simulink model "ROSCO"  (R2023a)
settings: Solver=ode4  StartTime=0.0  StopTime=TMax  FixedStep=simu.dt  RelTol=1e-3  EnableMultiTasking=on
undefined symbols (not defined in the file): A_total, Azimuth_list, B_total, Bd_total, C_total, D_total, Dd_total, DiscIntNeverNeededParam, F, n_FixFrameInputs, n_FixFrameOutputs, n_FixFrameStates2, n_RotTripletInputs, n_RotTripletOutputs, n_RotTripletStates2, new_seq_inp, new_seq_out, new_seq_states, OutList, Parameter, R, rpm2radps, simu, strmatch, uop_total, windspeed_list, wop_total, xop_total, yop_List_total
libraries: simulink x10
(part 1 of 5)
settings Model: Creator=nabbas  LastModifiedBy=16708
settings SolverCC: AlgebraicLoopSolver=TrustRegion
settings DataIOCC: SaveTime=off  ReturnWorkspaceOutputs=off  SignalLoggingName=sigsOut
settings DebuggingCC: UnconnectedInputMsg=warning  UnconnectedOutputMsg=warning  UnconnectedLineMsg=warning  ArithmeticOperatorsInVariantConditions=warning
settings ModelReferenceCC: EnableRefExpFcnMdlSchedulingChecks=on
settings SFSimCC: SimUseLocalCustomCode=off  CustomCodeUndefinedFunction=UseInterfaceOnly
settings RTWCC: RTWUseLocalCustomCode=off
settings CodeAppCC: StateflowObjectComments=on

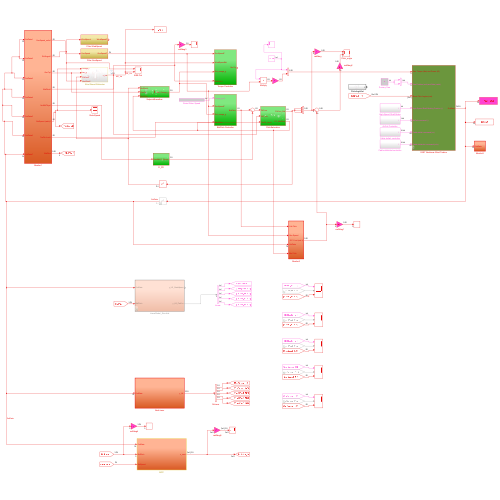
[thumbnail: Simulink's stored preview of the top-level diagram]
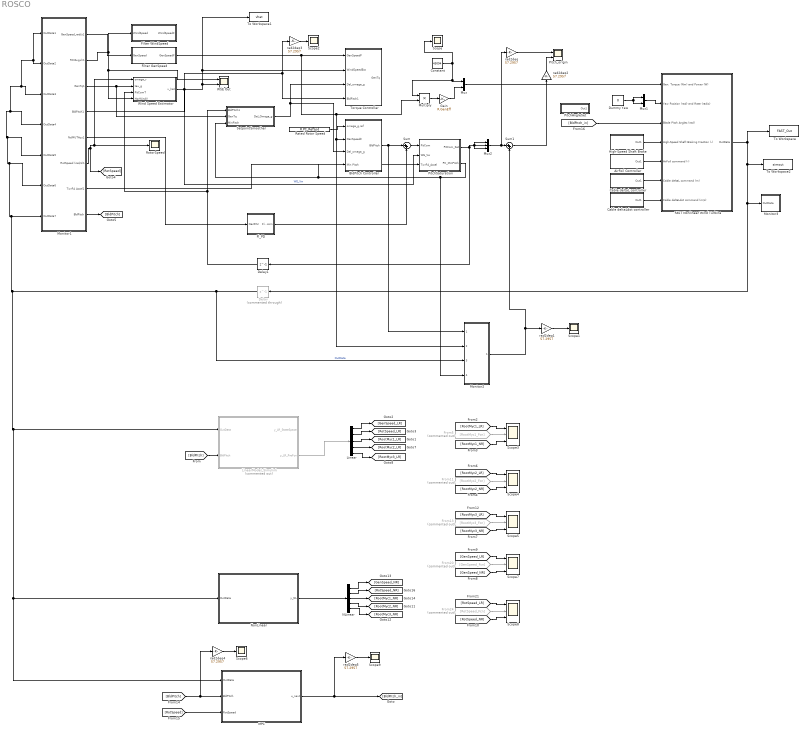
== system ROSCO ==
  AirFoil Controller : Subsystem
  BldPitch Controller : Subsystem
  Cable deltaL controller : Subsystem
  Cable deltaLdot controller : Subsystem
  Constant : Constant  Value=43094
  Delay : Delay  Commented=through  DelayLength=1
  Delay1 : Delay  DelayLength=1
  Dummy Yaw : Constant  Value=0
  FAST Nonlinear Wind Turbine : Subsystem  mask(FAST Nonlinear Wind Turbine){}
      mask help: This block contains the FAST S-Function.
      mask init:
      | clear FAST_SFunc
  Filter GenSpeed : Subsystem
  Filter WindSpeed : Subsystem
  Fl_PD : Subsystem
  From11 : From  Commented=on  GotoTag=RootMyc2_Fcn
  From13 : From  Commented=on  GotoTag=RootMyc3_Fcn
  From20 : From  Commented=on  GotoTag=GenSpeed_Fcn
  From24 : From  Commented=on  GotoTag=RotSpeed_Fcn
  From5 : From  Commented=on  GotoTag=RootMyc1_Fcn
  Gain : Gain  Gain=R.GenEff
  High-Speed Shaft Brake : Subsystem
  Linear : Demux  Outputs=5
  LinearModel_Simulink : Subsystem  Commented=on  TreatAsAtomicUnit=on
  MPC : Subsystem  TreatAsAtomicUnit=on
  Monitor1 : Subsystem  TreatAsAtomicUnit=on
  Monitor2 : Subsystem  TreatAsAtomicUnit=on
  Monitor3 : Subsystem  TreatAsAtomicUnit=on
  Multiply : Product
  Mux : Mux  Inputs=2
  Mux1 : Mux  Inputs=2
  Mux2 : Mux  Inputs=3
  NLinear : Demux  Outputs=5
  NonLinear : Subsystem  TreatAsAtomicUnit=on
  PitchAngleSet : Subsystem
  PitchSaturation : Subsystem
  Pitch_origin : Scope  NumInputPorts=2
  Rated Rotor Speed : Constant  Value=R.PC_RefSpd
  RotorSpeed : Scope
  Scope{,1..2,6,9} (5 alike) : Scope
  Scope{3..5,7..8} (5 alike) : Scope  NumInputPorts=3
  SetpointSmoother : Subsystem
  Sum : Sum  Inputs=|++
  Sum1 : Sum  Inputs=|++
  To Workspace : ToWorkspace  VariableName=FAST_Out  SaveFormat=Timeseries  SampleTime=-1
  To Workspace1 : ToWorkspace  VariableName=vhat  SaveFormat=Timeseries  SampleTime=-1
  To Workspace2 : ToWorkspace  VariableName=simout  SaveFormat=Timeseries  SampleTime=-1
  Torque Controller : Subsystem
  WSE Out : Scope  NumInputPorts=2
  Wind Speed Estimator : Subsystem
  rad2deg{,1..5} (6 alike) : Gain  Gain=57.2957
  wires:
  FAST Nonlinear Wind Turbine/1(OutData) -> To Workspace/1, To Workspace2/1, Monitor3/1(OutData), Delay/1
  Dummy Yaw/1 -> Mux1/2, Mux1/1
  Mux1/1 -> FAST Nonlinear Wind Turbine/2(Yaw Position (rad) and Rate (rad/s))
  Multiply/1 -> Gain/1
  Monitor1/1(GenSpeed_rad/s1) -> Filter GenSpeed/1(GenSpeed)
  Monitor1/3(GenTq1) -> SetpointSmoother/2(GenTq), Wind Speed Estimator/2(tau_g)
  SetpointSmoother/1(Del_Omega_g) -> BldPitch Controller/3(Del_omega_g), Torque Controller/3(Del_omega_g)
  Rated Rotor Speed/1 -> BldPitch Controller/1(omega_g,ref)
  Gain/1 -> Mux/2
  Monitor1/2(RtVAvgxh1) -> Wind Speed Estimator/4(HorWindV), WSE Out/1, Filter WindSpeed/1(WindSpeed)
  Wind Speed Estimator/1(v_hat) -> PitchSaturation/2(WE_Vw), WSE Out/2, Torque Controller/2(WindSpeedEst), To Workspace1/1  "WE_Vw"
  Monitor1/5(NcIMUTAys1) -> Fl_PD/1(NacIMU)
  Fl_PD/1(Fl_Pitcom) -> Sum/2
  Monitor1/4(BldPitch1) -> Torque Controller/4(BldPitch1), rad2deg3/1
  Sum/1 -> PitchSaturation/1(PitCom)
  PitchSaturation/1(PitCom_Sat) -> Delay1/1, Mux2/3, Mux2/1, Mux2/2
  PitchSaturation/2(PC_MinPitch) -> Monitor2/4(Min Pitch), BldPitch Controller/4(Min Pitch), SetpointSmoother/3(MinPitch)
  BldPitch Controller/1(BldPitch) -> Monitor2/1(Coll.Pitch), Sum/1
  Monitor1/6(RotSpeed (rad/s)1) -> [RotSpeed], RotorSpeed/1, Wind Speed Estimator/1(omega_r)
  Delay1/1 -> SetpointSmoother/1(BldPitch1), Wind Speed Estimator/3(PitComT)
  Monitor1/7(TwrFA Accel1) -> PitchSaturation/3(TwrFA_Accel)
  Mux/1 -> FAST Nonlinear Wind Turbine/1(Gen. Torque (Nm) and Power (W))
  Filter GenSpeed/1(GenSpeedF) -> Torque Controller/1(GenSpeedF), Multiply/2, Monitor2/2(Gen Speed), BldPitch Controller/2(GenSpeedF)
  Mux2/1 -> rad2deg/1, Sum1/1
  Sum1/1 -> rad2deg2/1
  High-Speed Shaft Brake/1(Out1) -> FAST Nonlinear Wind Turbine/4(High-Speed Shaft Braking Fraction (-))
  AirFoil Controller/1(Out1) -> FAST Nonlinear Wind Turbine/5(AirFoil command (-))
  Cable deltaL controller/1(Out1) -> FAST Nonlinear Wind Turbine/6(Cable deltaL command (m))
  Cable deltaLdot controller/1(Out1) -> FAST Nonlinear Wind Turbine/7(Cable deltaLdot command (m/s))
  rad2deg/1 -> Pitch_origin/1
  Monitor2/1(IPC Cmd (rad,3)) -> rad2deg1/1, Sum1/2
  rad2deg1/1 -> Scope1/1
  rad2deg2/1 -> Pitch_origin/2
  Constant/1 -> Scope/1, Multiply/1, Mux/1
  rad2deg3/1 -> Scope2/1
  [BldPitch] -> LinearModel_Simulink/2(BldPitch)
  Linear/5 -> [RootMyc3_LR]
  Linear/3 -> [RootMyc1_LR]
  Linear/2 -> [RotSpeed_LR]
  Linear/4 -> [RootMyc2_LR]
  Linear/1 -> [GenSpeed_LR]
  [RootMyc2_LR] -> Scope4/1
  From13/1 -> Scope5/2
  [RotSpeed_LR] -> Scope8/1
  [GenSpeed_LR] -> Scope7/1
  From11/1 -> Scope4/2
  From20/1 -> Scope7/2
  From5/1 -> Scope3/2
  [RootMyc3_LR] -> Scope5/1
  From24/1 -> Scope8/2
  [RootMyc1_LR] -> Scope3/1
  NLinear/3 -> [RootMyc1_NR]
  NonLinear/1(y_NL) -> NLinear/1
  NLinear/5 -> [RootMyc3_NR]
  NLinear/2 -> [RotSpeed_NR]
  NLinear/4 -> [RootMyc2_NR]
  NLinear/1 -> [GenSpeed_NR]
  [RootMyc1_NR] -> Scope3/3
  [RootMyc2_NR] -> Scope4/3
  [RootMyc3_NR] -> Scope5/3
  [GenSpeed_NR] -> Scope7/3
  [RotSpeed_NR] -> Scope8/3
  LinearModel_Simulink/2(y_LR_PreFcn) -> Linear/1
  [RotSpeed] -> MPC/3(RotSpeed)
  Delay/1 -> Monitor2/3(OutData), MPC/1(OutData), NonLinear/1(OutData), LinearModel_Simulink/1(OutData), Monitor1/4(OutData4), Monitor1/3(OutData3), Monitor1/1(OutData1), Monitor1/2(OutData2), Monitor1/5(OutData5), Monitor1/6(OutData6), Monitor1/7(OutData7)  "OutData"
  [BldPitch] -> rad2deg4/1, MPC/2(BldPitch)
  Monitor1/8(BldPitch) -> [BldPitch]
  rad2deg4/1 -> Scope6/1
  rad2deg5/1 -> Scope9/1
  MPC/1(u_next) -> rad2deg5/1, [BldPitch_in]
  [BldPitch_in] -> FAST Nonlinear Wind Turbine/3(Blade Pitch Angles (rad))

== system ROSCO/AirFoil Controller ==
  Airfoil command : Constant  Value=zeros(1,3)'
  Out1 : Outport
  wires:
  Airfoil command/1 -> Out1/1

== system ROSCO/BldPitch Controller ==
  note: % Cannot have "error pertubation" as control signal
      | - it is non-monotonic
  omega_g,ref : Inport
  GenSpeedF : Inport  Port=2
  Del_omega_g : Inport  Port=3
  Min Pitch : Inport  Port=4
  Compare To Zero1 : simulink/Logic and Bit Operations/Compare To Zero  relop=<  OutDataTypeStr=boolean
  Constant1 : Constant  Value=R.PC_GS_KP
  Constant2 : Constant  Value=R.PC_GS_KI
  Constant3 : Constant  Value=R.PC_GS_angles
  Delay : Delay  DelayLength=1
  Integral : Subsystem
  Multiply : Product
  Multiply3 : Product
  Mux : Mux  Inputs=5
  Pitch GS : MATLAB Function  TreatAsAtomicUnit=on
  Scope : Scope  Commented=on  NumInputPorts=2
  Scope1 : Scope  Commented=on
  Sum : Sum  Inputs=+-
  Sum1 : Sum  Inputs=|++
  Sum3 : Sum  Inputs=-+|
  To Workspace : ToWorkspace  VariableName=SpdErr  SaveFormat=Timeseries  SampleTime=-1
  To Workspace1 : ToWorkspace  VariableName=PC_params  SaveFormat=Structure  SampleTime=-1
  To Workspace2 : ToWorkspace  VariableName=Omega_bg_ref  SaveFormat=Timeseries  SampleTime=-1
  BldPitch : Outport  VectorParamsAs1DForOutWhenUnconnected=off
  wires:
  Multiply/1 -> Sum1/2
  Integral/1(IntSpdErr) -> Scope1/1, Sum1/1
  Pitch GS/1(Ki) -> Mux/3, Integral/2(Gain)
  Pitch GS/2(Kp) -> Mux/4, Multiply/2
  Mux/1 -> To Workspace1/1
  Sum1/1 -> Delay/1, BldPitch/1
  Sum3/1 -> Scope/1, To Workspace2/1, Sum/1
  GenSpeedF/1 -> Scope/2, Sum/2
  Compare To Zero1/1 -> Multiply3/1
  Del_omega_g/1 -> Compare To Zero1/1, Multiply3/2
  Multiply3/1 -> Sum3/1
  omega_g,ref/1 -> Sum3/2
  Constant1/1 -> Pitch GS/2(Kp_pc)
  Constant2/1 -> Pitch GS/3(Ki_pc)
  Constant3/1 -> Pitch GS/4(PC_beta)
  Delay/1 -> Pitch GS/1(Beta)
  Min Pitch/1 -> Integral/3(Min Pitch)
  Sum/1 -> To Workspace/1, Mux/2, Multiply/1, Integral/1(SpeedErr)

== system ROSCO/Cable deltaL controller ==
  Cable deltaL command : Constant  Value=zeros(1,20)'
  Out1 : Outport
  wires:
  Cable deltaL command/1 -> Out1/1

== system ROSCO/Cable deltaLdot controller ==
  Cable deltaLdot command : Constant  Value=zeros(1,20)'
  Out1 : Outport
  wires:
  Cable deltaLdot command/1 -> Out1/1

== system ROSCO/FAST Nonlinear Wind Turbine ==
  Gen. Torque (Nm) and Power (W) : Inport
  Yaw Position (rad) and Rate (rad/s) : Inport  Port=2
  Blade Pitch Angles (rad) : Inport  Port=3
  High-Speed Shaft Braking Fraction (-) : Inport  Port=4
  AirFoil command (-) : Inport  Port=5
  Cable deltaL command (m) : Inport  Port=6
  Cable deltaLdot command (m/s) : Inport  Port=7
  Mux1 : Mux  Inputs=7
  S-Function : S-Function  FunctionName=FAST_SFunc  Parameters=FAST_InputFileName, TMax, 0  SFunctionDeploymentMode=off  EnableBusSupport=off
  Signal Specification1 : SignalSpecification  OutDataTypeStr=double  Dimensions=2
  Signal Specification2 : SignalSpecification  OutDataTypeStr=double  Dimensions=2
  OutData : Outport
  wires:
  Gen. Torque (Nm) and Power (W)/1 -> Signal Specification1/1
  S-Function/1 -> OutData/1
  Mux1/1 -> S-Function/1
  Blade Pitch Angles (rad)/1 -> Mux1/3
  Yaw Position (rad) and Rate (rad/s)/1 -> Signal Specification2/1
  Signal Specification1/1 -> Mux1/1
  Signal Specification2/1 -> Mux1/2
  High-Speed Shaft Braking Fraction (-)/1 -> Mux1/4
  AirFoil command (-)/1 -> Mux1/5
  Cable deltaL command (m)/1 -> Mux1/6
  Cable deltaLdot command (m/s)/1 -> Mux1/7

== system ROSCO/Filter GenSpeed ==
  GenSpeed : Inport
  Discrete Filter : DiscreteFilter  Numerator=F.HSS.b  Denominator=F.HSS.a  InitialStates=R.VS_RefSpd/(sum(F.HSS.a(2:end))+1)
  Scope : Scope  NumInputPorts=2
  To Workspace2 : ToWorkspace  VariableName=Om_f  SaveFormat=Timeseries  SampleTime=-1
  GenSpeedF : Outport  VectorParamsAs1DForOutWhenUnconnected=off
  wires:
  Discrete Filter/1 -> Scope/2, To Workspace2/1, GenSpeedF/1
  GenSpeed/1 -> Scope/1, Discrete Filter/1

== system ROSCO/Filter WindSpeed ==
  WindSpeed : Inport
  Discrete Filter : DiscreteFilter  Numerator=F.Wind.b  Denominator=F.Wind.a  InitialStates=10
  To Workspace2 : ToWorkspace  VariableName=WindSpeedF  SaveFormat=Timeseries  SampleTime=-1
  WindSpeedF : Outport  VectorParamsAs1DForOutWhenUnconnected=off
  wires:
  Discrete Filter/1 -> WindSpeedF/1, To Workspace2/1
  WindSpeed/1 -> Discrete Filter/1

== system ROSCO/Fl_PD ==
  NacIMU : Inport
  Constant : Constant
  Enable : Gain  Gain=R.Fl_Mode
  Fl_HPF : DiscreteFilter  Numerator=F.F_Fl_HPF.b  Denominator=F.F_Fl_HPF.b
  Fl_LPF : DiscreteFilter  Numerator=F.F_Fl.b  Denominator=F.F_Fl.a
  Gain1 : Gain  Gain=-R.Fl_Kp
  Integral : Subsystem
  Scope : Scope
  Fl_Pitcom : Outport
  wires:
  Constant/1 -> Integral/2(Gain)
  NacIMU/1 -> Fl_LPF/1  "FA_AccR"
  Integral/1(Int x) -> Gain1/1
  Fl_HPF/1 -> Integral/1(x)  "FA_AccF"
  Gain1/1 -> Enable/1  "Fl_Pitcom"
  Enable/1 -> Scope/1, Fl_Pitcom/1  "Fl_Pitcom"
  Fl_LPF/1 -> Fl_HPF/1  "FA_AccF"

== system ROSCO/High-Speed Shaft Brake ==
  High-Speed Shaft Braking Fraction : Constant  Value=0
  Out1 : Outport
  wires:
  High-Speed Shaft Braking Fraction/1 -> Out1/1

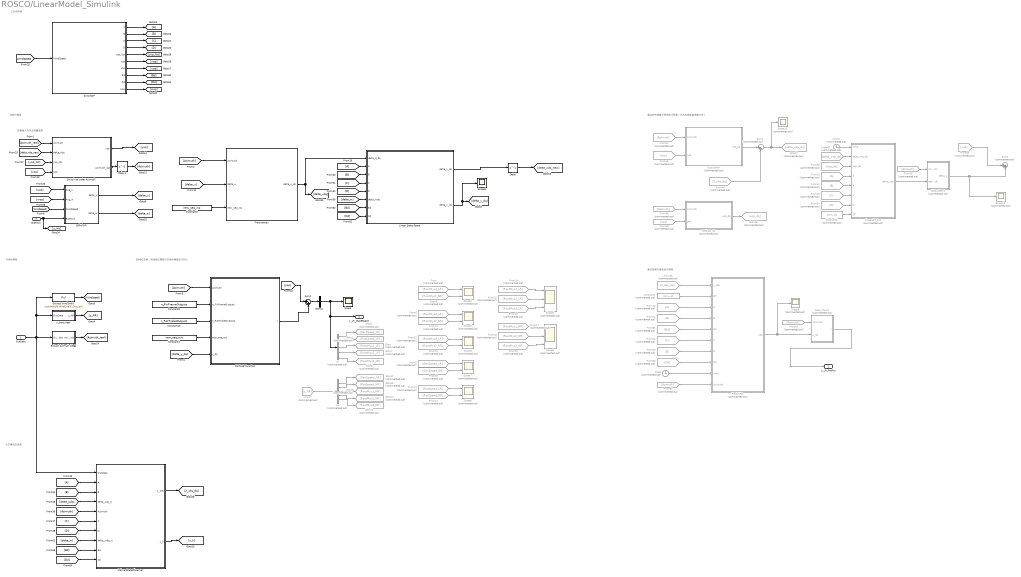
== system ROSCO/LinearModel_Simulink ==
  note: 通过时序递推方程来进行预测（无法应用数值求解方法）
  note: 通过预测方程来进行预测
  note: 卡尔曼状态观测
  note: 工作点转换
  note: 逆MBC变换，将线性化模型与非线性模型进行对比
  note: 控制输入与状态变量更新
  note: 线性化模型
  note: 非线性模型
  OutData : Inport
  BldPitch : Inport  Port=2
  Clock : Clock  Commented=on
  Clock1 : Clock  Commented=on
  Constant1 : Constant  Commented=on  Value=simu.dt
  Constant10 : Constant  Value=n_RotTripletOutputs
  Constant2 : Constant  Value=new_seq_inp
  Constant3 : Constant  Commented=on  Value=simu.dt
  Constant4 : Constant  Value=new_seq_out
  Constant9 : Constant  Value=n_FixFrameOutputs
  Delay : Delay  DelayLength=1  InitialCondition=0
  Delay1 : Delay  DelayLength=1  InitialCondition=0
  Demux : Demux  Outputs=1
  Diff of OP : MATLAB Function  TreatAsAtomicUnit=on
  Extract Azimuth [deg] : Subsystem
  Extract Wind1VelX : Fcn  Expr=u(strmatch('Wind1VelX',OutList))
  From : From  Commented=on  GotoTag=RootMyc1_LR
  From11 : From  Commented=on  GotoTag=RootMyc2_NR
  From12 : From  Commented=on  GotoTag=RootMyc3_LR
  From13 : From  Commented=on  GotoTag=RootMyc3_NR
  From14 : From  Commented=on  GotoTag=RootMyc1_LR
  From15 : From  Commented=on  GotoTag=RootMyc2_LR
  From16 : From  Commented=on  GotoTag=RootMyc3_LR
  From17 : From  Commented=on  GotoTag=RootMyc1_NR
  From18 : From  Commented=on  GotoTag=RootMyc2_NR
  From19 : From  Commented=on  GotoTag=RootMyc3_NR
  From20 : From  Commented=on  GotoTag=GenSpeed_NR
  From21 : From  Commented=on  GotoTag=RotSpeed_LR
  From24 : From  Commented=on  GotoTag=RotSpeed_NR
  From29 : From
  From33 : From
  From39 : From  Commented=on  GotoTag=X_obs_dq
  From40 : From  Commented=on
  From41 : From  Commented=on  GotoTag=B
  From42 : From  Commented=on  GotoTag=C
  From43 : From  Commented=on  GotoTag=D
  From{44,48,56..57,67} (5 alike) : From  Commented=on  GotoTag=Azimuth
  From45 : From  Commented=on  GotoTag=xop
  From46 : From  Commented=on  GotoTag=X_obs_dq
  From47 : From  Commented=on  GotoTag=delta_xop_dq
  From49 : From  Commented=on  GotoTag=uop
  From5 : From  Commented=on  GotoTag=RootMyc1_NR
  From50 : From  Commented=on  GotoTag=uop_dq
  From51 : From  Commented=on
  From52 : From  Commented=on  GotoTag=B
  From53 : From  Commented=on  GotoTag=C
  From54 : From  Commented=on  GotoTag=D
  From55 : From  Commented=on  GotoTag=yop
  From6 : From  Commented=on  GotoTag=RootMyc2_LR
  From65 : From  Commented=on  GotoTag=Bd
  From66 : From  Commented=on  GotoTag=Dd
  From7 : From  Commented=on  GotoTag=y_NR
  From9 : From  Commented=on  GotoTag=GenSpeed_LR
  Goto : Goto  Commented=on  GotoTag=RootMyc1_LR
  Goto1 : Goto  Commented=on  GotoTag=GenSpeed_LR
  Goto10 : Goto  Commented=on  GotoTag=RootMyc2_NR
  Goto11 : Goto  Commented=on  GotoTag=RootMyc3_NR
  Goto12 : Goto  Commented=on  GotoTag=GenSpeed_NR
  Goto16 : Goto  Commented=on  GotoTag=RotSpeed_NR
  Goto2 : Goto  Commented=on  GotoTag=RotSpeed_LR
  Goto23 : Goto
  Goto27 : Goto  Commented=on  GotoTag=delta_xop_dq
  Goto28 : Goto  Commented=on  GotoTag=uop_dq
  Goto7 : Goto  Commented=on  GotoTag=RootMyc2_LR
  Goto8 : Goto  Commented=on  GotoTag=RootMyc3_LR
  Goto9 : Goto  Commented=on  GotoTag=RootMyc1_NR
  KalmanStateObserver : Subsystem
  LR : Demux  Commented=on  Outputs=5
  Linear State-Space : Subsystem
  LinearWT_Fcn : MATLAB Function  Commented=on  TreatAsAtomicUnit=on
  MATLAB Function : MATLAB Function  TreatAsAtomicUnit=on
  NR : Demux  Commented=on  Outputs=5
  PredictFcn : MATLAB Function  Commented=on  TreatAsAtomicUnit=on
  Scope : Scope
  Scope{1..3,7..8} (5 alike) : Scope  Commented=on  NumInputPorts=2
  Scope10 : Scope  Commented=on
  Scope11 : Scope  Commented=on
  Scope4 : Scope  Commented=on  NumInputPorts=3
  Scope5 : Scope  Commented=on  NumInputPorts=3
  Scope6 : Scope
  Scope9 : Scope  Commented=on
  Subsystem : Subsystem  Commented=on
  Subsystem1 : Subsystem  Commented=on
  Subsystem2 : Subsystem  Commented=on
  Sum1 : Sum  Commented=on  Inputs=|-+
  Sum2 : Sum  Inputs=|++
  Sum3 : Sum  Commented=on  Inputs=|++
  Switch op under Azimuth : Subsystem
  SwitchOP : Subsystem
  Transverseu : Subsystem
  uop2uop_dq : Subsystem  Commented=on
  y_NonLinear : Subsystem
  y_LR_StateSpace : Outport
  y_LR_PreFcn : Outport  Port=2
  wires:
  OutData/1 -> Extract Azimuth [deg]/1(OutData), KalmanStateObserver/1(OutData), Extract Wind1VelX/1, y_NonLinear/1(OutData)
  Transverseu/1(delta_u_dq) -> [delta_udq], Linear State-Space/1(delta_u_dq)
  Demux/1 -> Scope/1, y_LR_StateSpace/1, LR/1
  y_NonLinear/1(y_NR) -> [y_NR]
  From7/1 -> NR/1
  Extract Wind1VelX/1 -> [WindSpeed]
  [Azimuth] -> Transverseu/1(Azimuth)
  Diff of OP/1(delta_u) -> [delta_u]
  [WindSpeed] -> Diff of OP/3(WindSpeed)
  [uop] -> Diff of OP/1(Avg_u)
  [delta_u] -> Transverseu/2(delta_u)
  Constant2/1 -> Transverseu/3(new_seq_inp)
  Constant9/1 -> MATLAB Function/2(n_FixFrameOutputs)
  Constant10/1 -> MATLAB Function/3(n_RotTripletOutputs)
  [Azimuth] -> MATLAB Function/1(Azimuth)
  Constant4/1 -> MATLAB Function/4(new_seq_out)
  LR/3 -> Goto/1
  LR/4 -> Goto7/1
  LR/5 -> Goto8/1
  NR/3 -> Goto9/1
  NR/4 -> Goto10/1
  NR/5 -> Goto11/1
  From/1 -> Scope1/1
  From5/1 -> Scope1/2
  From6/1 -> Scope2/1
  From11/1 -> Scope2/2
  From12/1 -> Scope3/1
  From13/1 -> Scope3/2
  From14/1 -> Scope4/1
  From15/1 -> Scope4/2
  From16/1 -> Scope4/3
  From17/1 -> Scope5/1
  From18/1 -> Scope5/2
  From19/1 -> Scope5/3
  Linear State-Space/1(delta_x_dq) -> Delay/1
  Switch op under Azimuth/1(yop) -> [yop]
  [Azimuth_real] -> Switch op under Azimuth/1(Azimuth)
  [yop] -> Sum2/1
  Linear State-Space/2(delta_y_dq) -> Scope6/1, [delta_y_dq]
  Delay/1 -> [delta_xdq_new]
  Switch op under Azimuth/2(Azimuth_out) -> Delay1/1
  Delay1/1 -> [Azimuth]
  [delta_xdq_new] -> Switch op under Azimuth/2(delta_xdq)
  LR/1 -> Goto1/1
  LR/2 -> Goto2/1
  NR/1 -> Goto12/1
  NR/2 -> Goto16/1
  From9/1 -> Scope7/1
  From20/1 -> Scope7/2
  From21/1 -> Scope8/1
  From24/1 -> Scope8/2
  BldPitch/1 -> [u_init], Diff of OP/4(BldPitch)
  [WindSpeed] -> SwitchOP/1(WindSpeed)
  SwitchOP/7(uop) -> [uop]
  SwitchOP/6(xop) -> [xop]
  SwitchOP/5(yop_list) -> [yop_list]
  SwitchOP/4(D) -> [D]
  SwitchOP/3(C) -> [C]
  SwitchOP/2(B) -> [B]
  SwitchOP/1(A) -> Goto23/1
  [yop_list] -> Switch op under Azimuth/3(yop_list)
  [xop] -> Switch op under Azimuth/4(xop)
  From29/1 -> Linear State-Space/2(A)
  [B] -> Linear State-Space/3(B)
  [C] -> Linear State-Space/4(C)
  [D] -> Linear State-Space/5(D)
  Extract Azimuth [deg]/1(Azimuth) -> [Azimuth_real]
  [delta_y_dq] -> MATLAB Function/5(y_dq)
  MATLAB Function/1(y) -> Sum2/2
  Sum2/1 -> Demux/1
  From33/1 -> KalmanStateObserver/2(A)
  [B] -> KalmanStateObserver/3(B)
  [delta_udq] -> KalmanStateObserver/4(delta_udq_in)
  [C] -> KalmanStateObserver/6(C)
  [D] -> KalmanStateObserver/7(D)
  [Azimuth] -> KalmanStateObserver/5(Azimuth)
  KalmanStateObserver/1(X_obs) -> [X_obs_dq]
  Constant1/1 -> PredictFcn/2(DT)
  From39/1 -> PredictFcn/1(x_obs)
  From40/1 -> PredictFcn/3(A)
  From41/1 -> PredictFcn/4(B)
  From42/1 -> PredictFcn/6(C)
  From43/1 -> PredictFcn/7(D)
  Clock/1 -> PredictFcn/9(time)
  From44/1 -> Subsystem/1(Azimuth)
  From45/1 -> Subsystem/2(xop)
  Subsystem/1(xop_dq) -> Sum1/1
  From46/1 -> Sum1/2
  Sum1/1 -> Goto27/1, Scope10/1
  Clock1/1 -> LinearWT_Fcn/1(time)
  From47/1 -> LinearWT_Fcn/2(delta_xop_dq)
  From48/1 -> uop2uop_dq/1(Azimuth)
  From49/1 -> uop2uop_dq/2(uop)
  uop2uop_dq/1(uop_dq) -> Goto28/1
  From50/1 -> LinearWT_Fcn/3(uop_dq)
  From51/1 -> LinearWT_Fcn/4(A)
  From52/1 -> LinearWT_Fcn/5(B)
  From53/1 -> LinearWT_Fcn/6(C)
  From54/1 -> LinearWT_Fcn/7(D)
  Constant3/1 -> LinearWT_Fcn/8(DT)
  From55/1 -> Sum3/1
  Subsystem1/1(delta_y) -> Scope11/1, Sum3/2
  LinearWT_Fcn/1(delta_ydq) -> Subsystem1/2(delta_y_dq)
  From56/1 -> Subsystem1/1(Azimuth)
  From57/1 -> Subsystem2/1(Azimuth)
  PredictFcn/1(ydq) -> Scope9/1, Subsystem2/2(y_dq)
  Subsystem2/1(y) -> y_LR_PreFcn/1
  KalmanStateObserver/2(x_k) -> [x_k]
  SwitchOP/8(Bd) -> [Bd]
  SwitchOP/9(Dd) -> [Dd]
  SwitchOP/10(wop) -> [wop]
  [wop] -> Diff of OP/2(Avg_w)
  Diff of OP/2(delta_w) -> [delta_w]
  [Bd] -> Linear State-Space/7(Bd)
  [delta_w] -> Linear State-Space/6(delta_wdq)
  [Dd] -> Linear State-Space/8(Dd)
  [delta_w] -> KalmanStateObserver/8(delta_wdq_in)
  [Bd] -> KalmanStateObserver/9(Bd)
  [Dd] -> KalmanStateObserver/10(Dd)
  From65/1 -> PredictFcn/5(Bd)
  From66/1 -> PredictFcn/8(Dd)
  From67/1 -> PredictFcn/10(Azimuth)

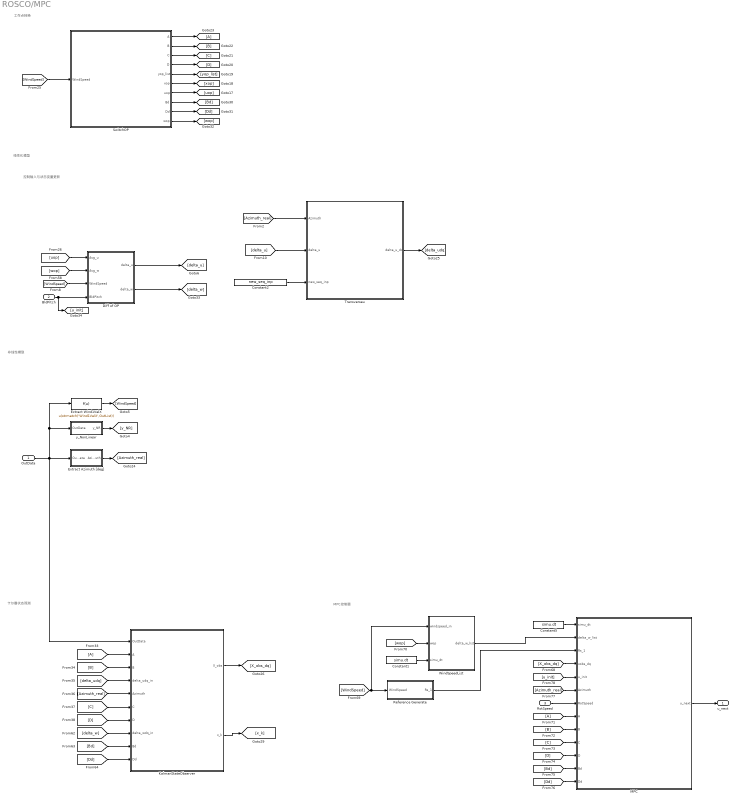
== system ROSCO/MPC ==
  note: MPC控制器
  note: 卡尔曼状态观测
  note: 工作点转换
  note: 控制输入与状态变量更新
  note: 线性化模型
  note: 非线性模型
  OutData : Inport
  BldPitch : Inport  Port=2
  RotSpeed : Inport  Port=3
  Constant1 : Constant  Value=simu.dt
  Constant2 : Constant  Value=new_seq_inp
  Constant5 : Constant  Value=simu.dt
  Diff of OP : MATLAB Function  TreatAsAtomicUnit=on
  Extract Azimuth [deg] : Subsystem
  Extract Wind1VelX : Fcn  Expr=u(strmatch('Wind1VelX',OutList))
  From33 : From
  From71 : From
  Goto23 : Goto
  KalmanStateObserver : Subsystem
  MPC : MATLAB Function  TreatAsAtomicUnit=on
  Reference Generate : MATLAB Function  TreatAsAtomicUnit=on
  SwitchOP : Subsystem
  Transverseu : Subsystem
  WindSpeedList : MATLAB Function  TreatAsAtomicUnit=on
  y_NonLinear : Subsystem
  u_next : Outport
  wires:
  OutData/1 -> Extract Azimuth [deg]/1(OutData), KalmanStateObserver/1(OutData), Extract Wind1VelX/1, y_NonLinear/1(OutData)
  Transverseu/1(delta_u_dq) -> [delta_udq]
  y_NonLinear/1(y_NR) -> [y_NR]
  Extract Wind1VelX/1 -> [WindSpeed]
  [Azimuth_real] -> Transverseu/1(Azimuth)
  Diff of OP/1(delta_u) -> [delta_u]
  [WindSpeed] -> Diff of OP/3(WindSpeed)
  [uop] -> Diff of OP/1(Avg_u)
  [delta_u] -> Transverseu/2(delta_u)
  Constant2/1 -> Transverseu/3(new_seq_inp)
  BldPitch/1 -> [u_init], Diff of OP/4(BldPitch)
  [WindSpeed] -> SwitchOP/1(WindSpeed)
  SwitchOP/7(uop) -> [uop]
  SwitchOP/6(xop) -> [xop]
  SwitchOP/5(yop_list) -> [yop_list]
  SwitchOP/4(D) -> [D]
  SwitchOP/3(C) -> [C]
  SwitchOP/2(B) -> [B]
  SwitchOP/1(A) -> Goto23/1
  Extract Azimuth [deg]/1(Azimuth) -> [Azimuth_real]
  From33/1 -> KalmanStateObserver/2(A)
  [B] -> KalmanStateObserver/3(B)
  [delta_udq] -> KalmanStateObserver/4(delta_udq_in)
  [C] -> KalmanStateObserver/6(C)
  [D] -> KalmanStateObserver/7(D)
  [Azimuth_real] -> KalmanStateObserver/5(Azimuth)
  KalmanStateObserver/1(X_obs) -> [X_obs_dq]
  KalmanStateObserver/2(x_k) -> [x_k]
  SwitchOP/8(Bd) -> [Bd]
  SwitchOP/9(Dd) -> [Dd]
  SwitchOP/10(wop) -> [wop]
  [wop] -> Diff of OP/2(Avg_w)
  Diff of OP/2(delta_w) -> [delta_w]
  [delta_w] -> KalmanStateObserver/8(delta_wdq_in)
  [Bd] -> KalmanStateObserver/9(Bd)
  [Dd] -> KalmanStateObserver/10(Dd)
  MPC/1(u_next) -> u_next/1
  Constant5/1 -> MPC/1(simu_dt)
  [X_obs_dq] -> MPC/4(xobs_dq)
  [WindSpeed] -> WindSpeedList/1(windspeed_in), Reference Generate/1(WindSpeed)
  [wop] -> WindSpeedList/2(wop)
  From71/1 -> MPC/8(A)
  [B] -> MPC/9(B)
  [C] -> MPC/10(C)
  [D] -> MPC/11(D)
  [Bd] -> MPC/12(Bd)
  [Dd] -> MPC/13(Dd)
  [Azimuth_real] -> MPC/6(Azimuth)
  RotSpeed/1 -> MPC/7(RotSpeed)
  [u_init] -> MPC/5(u_init)
  WindSpeedList/1(delta_w_list) -> MPC/2(delta_w_list)
  Constant1/1 -> WindSpeedList/3(simu_dt)
  Reference Generate/1(Rs_1) -> MPC/3(Rs_1)

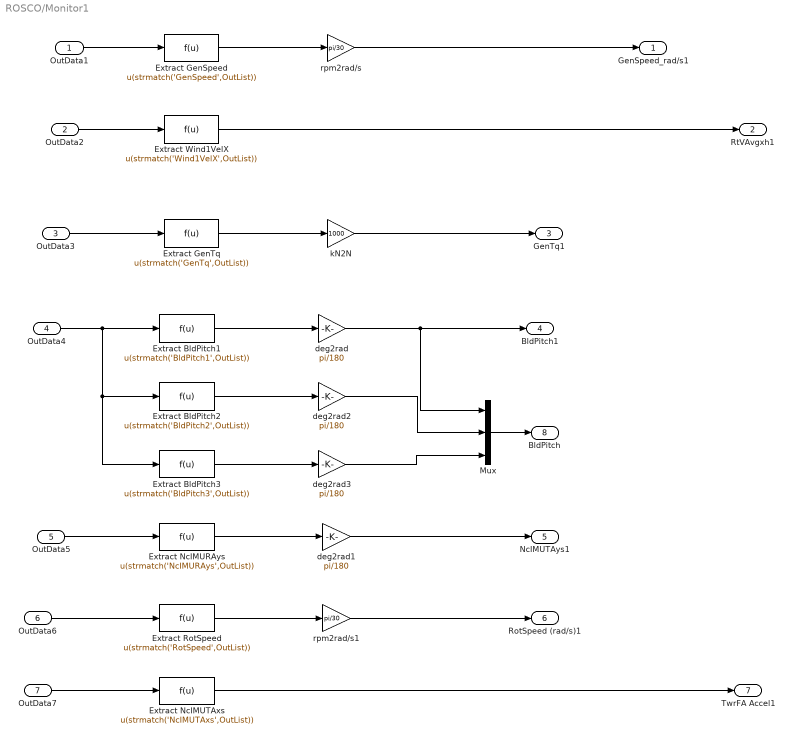
== system ROSCO/Monitor1 ==
  OutData1 : Inport
  OutData2 : Inport  Port=2
  OutData3 : Inport  Port=3
  OutData4 : Inport  Port=4
  OutData5 : Inport  Port=5
  OutData6 : Inport  Port=6
  OutData7 : Inport  Port=7
  Extract BldPitch1 : Fcn  Expr=u(strmatch('BldPitch1',OutList))
  Extract BldPitch2 : Fcn  Expr=u(strmatch('BldPitch2',OutList))
  Extract BldPitch3 : Fcn  Expr=u(strmatch('BldPitch3',OutList))
  Extract GenSpeed : Fcn  Expr=u(strmatch('GenSpeed',OutList))
  Extract GenTq : Fcn  Expr=u(strmatch('GenTq',OutList))
  Extract NcIMURAys : Fcn  Expr=u(strmatch('NcIMURAys',OutList))
  Extract NcIMUTAxs : Fcn  Expr=u(strmatch('NcIMUTAxs',OutList))
  Extract RotSpeed : Fcn  Expr=u(strmatch('RotSpeed',OutList))
  Extract Wind1VelX : Fcn  Expr=u(strmatch('Wind1VelX',OutList))
  Mux : Mux  Inputs=3
  deg2rad{,1..3} (4 alike) : Gain  Gain=pi/180
  kN2N : Gain  Gain=1000
  rpm2rad/s : Gain  Gain=pi/30
  rpm2rad/s1 : Gain  Gain=pi/30
  GenSpeed_rad/s1 : Outport  VectorParamsAs1DForOutWhenUnconnected=off
  RtVAvgxh1 : Outport  Port=2  VectorParamsAs1DForOutWhenUnconnected=off
  GenTq1 : Outport  Port=3  VectorParamsAs1DForOutWhenUnconnected=off
  BldPitch1 : Outport  Port=4  VectorParamsAs1DForOutWhenUnconnected=off
  NcIMUTAys1 : Outport  Port=5  VectorParamsAs1DForOutWhenUnconnected=off
  RotSpeed (rad/s)1 : Outport  Port=6  VectorParamsAs1DForOutWhenUnconnected=off
  TwrFA Accel1 : Outport  Port=7  VectorParamsAs1DForOutWhenUnconnected=off
  BldPitch : Outport  Port=8  VectorParamsAs1DForOutWhenUnconnected=off
  wires:
  Extract NcIMURAys/1 -> deg2rad1/1
  Extract GenSpeed/1 -> rpm2rad/s/1
  OutData5/1 -> Extract NcIMURAys/1
  Extract NcIMUTAxs/1 -> TwrFA Accel1/1
  rpm2rad/s1/1 -> RotSpeed (rad/s)1/1
  Extract RotSpeed/1 -> rpm2rad/s1/1
  Extract BldPitch1/1 -> deg2rad/1
  rpm2rad/s/1 -> GenSpeed_rad/s1/1
  OutData3/1 -> Extract GenTq/1
  deg2rad1/1 -> NcIMUTAys1/1
  kN2N/1 -> GenTq1/1
  OutData7/1 -> Extract NcIMUTAxs/1
  deg2rad/1 -> Mux/1, BldPitch1/1
  OutData2/1 -> Extract Wind1VelX/1
  Extract GenTq/1 -> kN2N/1
  Extract Wind1VelX/1 -> RtVAvgxh1/1
  OutData1/1 -> Extract GenSpeed/1
  OutData6/1 -> Extract RotSpeed/1
  Extract BldPitch2/1 -> deg2rad2/1
  Extract BldPitch3/1 -> deg2rad3/1
  OutData4/1 -> Extract BldPitch2/1, Extract BldPitch3/1, Extract BldPitch1/1
  deg2rad2/1 -> Mux/2
  deg2rad3/1 -> Mux/3
  Mux/1 -> BldPitch/1

== system ROSCO/Monitor2 ==
  Coll.Pitch : Inport
  Gen Speed : Inport  Port=2
  OutData : Inport  Port=3
  Min Pitch : Inport  Port=4
  Cyclic Pitch controller : Subsystem  TreatAsAtomicUnit=on
      settings: MinAlgLoopOccurrences=on
  IPC Cmd (rad,3) : Outport
  wires:
  Min Pitch/1 -> Cyclic Pitch controller/4(Min PItch (rad))
  Coll.Pitch/1 -> Cyclic Pitch controller/1(Coll. Pitch)
  Cyclic Pitch controller/1(IPC Cmd (rad,3)) -> IPC Cmd (rad,3)/1
  Gen Speed/1 -> Cyclic Pitch controller/2(Gen Speed)
  OutData/1 -> Cyclic Pitch controller/3(OutData)

== system ROSCO/Monitor3 ==
  OutData : Inport
  Extract BldPitch1 : Fcn  Expr=u(strmatch('BldPitch1',OutList))
  Extract GenPwr : Fcn  Expr=u(strmatch('GenPwr',OutList))
  Extract GenTq : Fcn  Expr=u(strmatch('GenTq',OutList))
  Extract RotSpeed : Fcn  Expr=u(strmatch('RotSpeed',OutList))
  Scope : Scope  NumInputPorts=4
  Scope1 : Scope
  wires:
  OutData/1 -> Extract RotSpeed/1, Extract GenPwr/1, Extract BldPitch1/1, Extract GenTq/1
  Extract GenPwr/1 -> Scope1/1, Scope/4
  Extract GenTq/1 -> Scope/2
  Extract BldPitch1/1 -> Scope/3
  Extract RotSpeed/1 -> Scope/1

== system ROSCO/NonLinear ==
  OutData : Inport
  Extract GenSpeed : Fcn  Expr=u(strmatch('GenSpeed',OutList))
  Extract RootMyc1 : Fcn  Expr=u(strmatch('RootMyc1',OutList))
  Extract RootMyc2 : Fcn  Expr=u(strmatch('RootMyc2',OutList))
  Extract RootMyc3 : Fcn  Expr=u(strmatch('RootMyc3',OutList))
  Extract RotSpeed : Fcn  Expr=u(strmatch('RotSpeed',OutList))
  Mux : Mux  Inputs=5
  y_NL : Outport
  wires:
  Extract RotSpeed/1 -> Mux/2
  Extract GenSpeed/1 -> Mux/1
  Mux/1 -> y_NL/1
  OutData/1 -> Extract GenSpeed/1, Extract RotSpeed/1, Extract RootMyc2/1, Extract RootMyc3/1, Extract RootMyc1/1
  Extract RootMyc1/1 -> Mux/3
  Extract RootMyc2/1 -> Mux/4
  Extract RootMyc3/1 -> Mux/5

== system ROSCO/PitchAngleSet ==
  Blade Pitch Angles [deg] : Constant  Value=8.42
  Blade Pitch Angles [deg]1 : Constant  Value=8.42
  Blade Pitch Angles [deg]2 : Constant  Value=8.42
  Mux3 : Mux  Inputs=3
  Step : Step  Time=100  SampleTime=0
  Step1 : Step  Time=100  After=-1  SampleTime=0
  Step2 : Step  Time=100  SampleTime=0
  Sum1 : Sum  Inputs=|++
  Sum2 : Sum  Inputs=|++
  Sum3 : Sum  Inputs=|++
  deg2rad : Gain  Gain=1/(57.2957)
  deg2rad1 : Gain  Gain=1/(57.2957)
  deg2rad2 : Gain  Gain=1/(57.2957)
  Out1 : Outport
  wires:
  Blade Pitch Angles [deg]/1 -> Sum2/1
  Sum2/1 -> deg2rad/1
  Mux3/1 -> Out1/1
  Step/1 -> Sum2/2
  deg2rad/1 -> Mux3/1
  Sum1/1 -> deg2rad1/1
  deg2rad1/1 -> Mux3/2
  Blade Pitch Angles [deg]1/1 -> Sum1/1
  Step1/1 -> Sum1/2
  Sum3/1 -> deg2rad2/1
  deg2rad2/1 -> Mux3/3
  Blade Pitch Angles [deg]2/1 -> Sum3/1
  Step2/1 -> Sum3/2

== system ROSCO/PitchSaturation ==
  note: 输出桨距角下限
  note: 根据等效风速确定桨距角下限
  PitCom : Inport
  WE_Vw : Inport  Port=2
  TwrFA_Accel : Inport  Port=3
  1-D Lookup Table : Lookup_n-D  NumberOfTableDimensions=1  BreakpointsForDimension1=R.PS_WindSpeeds  Table=R.PS_BldPitchMin  InternalRulePriority=Speed  RndMeth=Simplest
  Constant : Constant  Value=R.PS_Mode
  Constant1 : Constant  Value=R.PC_MinPit
  Constant2 : Constant
  Constant4 : Constant  Value=R.PC_MaxPit
  Discrete Filter : DiscreteFilter  Numerator=F.F_PS.b  Denominator=F.F_PS.a  InitialStates=R.WE_v0/(sum(F.F_PS.a(2:end))+1)
  Integral : Subsystem
  Mux : Mux  Inputs=2
  Rate Limiter1 : RateLimiter  RisingSlewLimit=R.PC_MaxRat  FallingSlewLimit=-R.PC_MaxRat  SampleTimeMode=inherited
  Scope : Scope  Commented=on  NumInputPorts=3
  Scope1 : Scope  Commented=on  NumInputPorts=3
  Sum : Sum  Inputs=|++
  Switch : Switch  Criteria=u2 > Threshold  Threshold=0.5  SaturateOnIntegerOverflow=off  InputSameDT=off
  Variable Saturator1 : MATLAB Function  TreatAsAtomicUnit=on
  PitCom_Sat : Outport
  PC_MinPitch : Outport  Port=2
  wires:
  1-D Lookup Table/1 -> Scope/3, Switch/1
  Constant/1 -> Switch/2
  Discrete Filter/1 -> Scope/2, 1-D Lookup Table/1  "Vhatf"
  Constant1/1 -> Switch/3
  Switch/1 -> PC_MinPitch/1, Variable Saturator1/2(lowerLimit)  "PC_MinPit"
  Constant4/1 -> Variable Saturator1/3(upperLimit)
  Variable Saturator1/1(pitchCommandOut) -> Scope1/1, Rate Limiter1/1
  Rate Limiter1/1 -> Scope1/2, PitCom_Sat/1
  PitCom/1 -> Variable Saturator1/1(pitchCommand)
  TwrFA_Accel/1 -> Integral/1(x)
  Constant2/1 -> Integral/2(Gain)
  WE_Vw/1 -> Mux/1, Sum/1
  Sum/1 -> Mux/2, Discrete Filter/1
  Mux/1 -> Scope/1

== system ROSCO/SetpointSmoother ==
  BldPitch1 : Inport
  GenTq : Inport  Port=2
  MinPitch : Inport  Port=3
  Constant : Constant  Value=R.PC_MinPit
  Constant1 : Constant  Value=R.SS_VSGain
  Constant2 : Constant  Value=R.VS_RtTq
  Constant3 : Constant  Value=R.SS_PCGain
  Divide : Product  Inputs=**
  Divide1 : Product  Inputs=**
  Filter Delta_GenRef : Subsystem
  Gain : Gain  Gain=1/deg2rad(30)
  Gain1 : Gain  Gain=1/R.VS_RtTq
  Gain2 : Gain  Gain=R.VS_RefSpd
  Sum : Sum  Inputs=|+-
  Sum1 : Sum  Inputs=+-|
  Sum2 : Sum  Inputs=+|-
  To Workspace : ToWorkspace  VariableName=DelOmega  SaveFormat=Timeseries  SampleTime=-1
  To Workspace1 : ToWorkspace  VariableName=BldPitch_GB  SaveFormat=Timeseries  SampleTime=-1
  To Workspace2 : ToWorkspace  VariableName=Torque_GB  SaveFormat=Timeseries  SampleTime=-1
  Del_Omega_g : Outport  VectorParamsAs1DForOutWhenUnconnected=off
  wires:
  Divide1/1 -> Sum2/2, To Workspace2/1
  Divide/1 -> Sum2/1, To Workspace1/1
  Filter Delta_GenRef/1(GainBiasF) -> Gain2/1
  Constant3/1 -> Divide1/1
  Constant1/1 -> Divide/2
  Sum/1 -> Gain/1
  BldPitch1/1 -> Sum/1
  Sum2/1 -> Filter Delta_GenRef/1(GainBias)
  Constant2/1 -> Sum1/1
  Sum1/1 -> Gain1/1
  GenTq/1 -> Sum1/2
  Gain/1 -> Divide/1
  Gain1/1 -> Divide1/2
  Gain2/1 -> To Workspace/1, Del_Omega_g/1  "SS_DelOmegaF"
  Constant/1 -> Sum/2

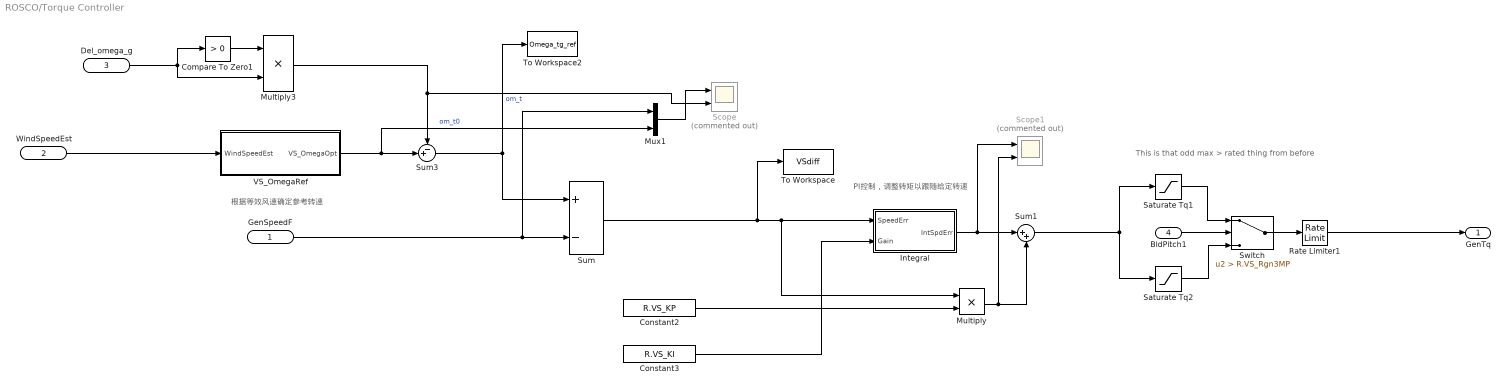
== system ROSCO/Torque Controller ==
  note: PI控制，调整转矩以跟随给定转速
  note: 根据等效风速确定参考转速
  note: This is that odd max > rated thing from before
  GenSpeedF : Inport
  WindSpeedEst : Inport  Port=2
  Del_omega_g : Inport  Port=3
  BldPitch1 : Inport  Port=4
  Compare To Zero1 : simulink/Logic and Bit Operations/Compare To Zero  relop=>  OutDataTypeStr=boolean
  Constant2 : Constant  Value=R.VS_KP
  Constant3 : Constant  Value=R.VS_KI
  Integral : Subsystem
  Multiply : Product
  Multiply3 : Product
  Mux1 : Mux  Inputs=2
  Rate Limiter1 : RateLimiter  RisingSlewLimit=R.VS_MaxRat  FallingSlewLimit=-R.VS_MaxRat  SampleTimeMode=inherited  InitialCondition=R.VS_RtTq
  Saturate Tq1 : Saturate  UpperLimit=R.VS_RtTq  LowerLimit=0
  Saturate Tq2 : Saturate  UpperLimit=R.VS_RtTq  LowerLimit=0
  Scope : Scope  Commented=on  NumInputPorts=2
  Scope1 : Scope  Commented=on  NumInputPorts=2
  Sum : Sum  Inputs=+-
  Sum1 : Sum  Inputs=|++
  Sum3 : Sum  Inputs=-+|
  Switch : Switch  Criteria=u2 > Threshold  Threshold=R.VS_Rgn3MP  SaturateOnIntegerOverflow=off  InputSameDT=off
  To Workspace : ToWorkspace  VariableName=VSdiff  SaveFormat=Timeseries  SampleTime=-1
  To Workspace2 : ToWorkspace  VariableName=Omega_tg_ref  SaveFormat=Timeseries  SampleTime=-1
  VS_OmegaRef : Subsystem
  GenTq : Outport  VectorParamsAs1DForOutWhenUnconnected=off
  wires:
  Multiply/1 -> Scope1/2, Sum1/2
  Integral/1(IntSpdErr) -> Scope1/1, Sum1/1
  Constant2/1 -> Multiply/2
  Constant3/1 -> Integral/2(Gain)
  VS_OmegaRef/1(VS_OmegaOpt) -> Mux1/2, Sum3/2  "om_t0"
  GenSpeedF/1 -> Mux1/1, Sum/2
  Sum3/1 -> To Workspace2/1, Sum/1  "om_t"
  Saturate Tq2/1 -> Switch/3
  Switch/1 -> Rate Limiter1/1
  Saturate Tq1/1 -> Switch/1
  BldPitch1/1 -> Switch/2
  Compare To Zero1/1 -> Multiply3/1
  Del_omega_g/1 -> Compare To Zero1/1, Multiply3/2
  Multiply3/1 -> Scope/2, Sum3/1
  Mux1/1 -> Scope/1
  Sum1/1 -> Saturate Tq2/1, Saturate Tq1/1
  Rate Limiter1/1 -> GenTq/1
  Sum/1 -> To Workspace/1, Integral/1(SpeedErr), Multiply/1
  WindSpeedEst/1 -> VS_OmegaRef/1(WindSpeedEst)

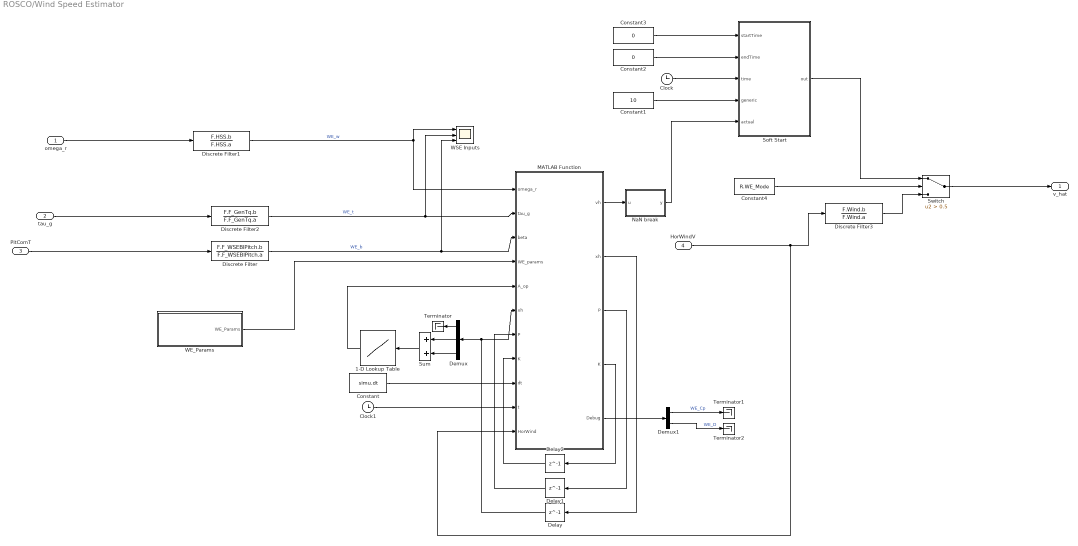
== system ROSCO/Wind Speed Estimator ==
  omega_r : Inport
  tau_g : Inport  Port=2
  PitComT : Inport  Port=3
  HorWindV : Inport  Port=4
  1-D Lookup Table : Lookup_n-D  NumberOfTableDimensions=1  BreakpointsForDimension1=[-5:5]  Table=tanh([-5:5])  InternalRulePriority=Speed  RndMeth=Simplest
  Clock : Clock
  Clock1 : Clock
  Constant : Constant  Value=simu.dt
  Constant1 : Constant  Value=10
  Constant2 : Constant  Value=0
  Constant3 : Constant  Value=0
  Constant4 : Constant  Value=R.WE_Mode
  Delay : Delay  DelayLength=1  InitialCondition=[R.WE_GearboxRatio, 0, R.WE_v0]'
  Delay1 : Delay  DelayLength=1  InitialCondition=diag([0.1, 0.1, 1])^2
  Delay2 : Delay  DelayLength=1  InitialCondition=zeros(3,1)
  Demux : Demux  Outputs=3
  Demux1 : Demux  Outputs=2
  Discrete Filter : DiscreteFilter  Numerator=F.F_WSEBlPitch.b  Denominator=F.F_WSEBlPitch.a
  Discrete Filter1 : DiscreteFilter  Numerator=F.HSS.b  Denominator=F.HSS.a  InitialStates=R.VS_RefSpd/(sum(F.HSS.a(2:end))+1)/R.GBRatio
  Discrete Filter2 : DiscreteFilter  Numerator=F.F_GenTq.b  Denominator=F.F_GenTq.a  InitialStates=R.VS_RtTq/(sum(F.F_GenTq.a(2:end))+1)
  Discrete Filter3 : DiscreteFilter  Numerator=F.Wind.b  Denominator=F.Wind.a  InitialStates=10
  MATLAB Function : MATLAB Function  TreatAsAtomicUnit=on
  NaN break : MATLAB Function  TreatAsAtomicUnit=on
  Soft Start : MATLAB Function  TreatAsAtomicUnit=on
  Sum : Sum
  Switch : Switch  Criteria=u2 > Threshold  Threshold=0.5  SaturateOnIntegerOverflow=off  InputSameDT=off
  Terminator : Terminator
  Terminator1 : Terminator
  Terminator2 : Terminator
  WE_Params : Subsystem
  WSE Inputs : Scope  NumInputPorts=3
  v_hat : Outport  VectorParamsAs1DForOutWhenUnconnected=off
  wires:
  MATLAB Function/2(xh) -> Delay/1
  Delay/1 -> Demux/1, MATLAB Function/6("xh ")
  MATLAB Function/3(P) -> Delay1/1
  Delay1/1 -> MATLAB Function/7("P ")
  omega_r/1 -> Discrete Filter1/1
  tau_g/1 -> Discrete Filter2/1
  MATLAB Function/4(K) -> Delay2/1
  Delay2/1 -> MATLAB Function/8("K ")
  Constant/1 -> MATLAB Function/9(dt)
  Demux/2 -> Sum/1
  Demux/3 -> Sum/2
  Demux/1 -> Terminator/1
  Sum/1 -> 1-D Lookup Table/1
  1-D Lookup Table/1 -> MATLAB Function/5(A_op)
  WE_Params/1(WE_Params) -> MATLAB Function/4(WE_params)
  Clock/1 -> Soft Start/3(time)
  Constant1/1 -> Soft Start/4(generic)
  Constant2/1 -> Soft Start/2(endTime)
  Constant3/1 -> Soft Start/1(startTime)
  MATLAB Function/1(vh) -> NaN break/1(u)
  Discrete Filter/1 -> WSE Inputs/3, MATLAB Function/3(beta)  "WE_b"
  Discrete Filter1/1 -> MATLAB Function/1(omega_r), WSE Inputs/1  "WE_w"
  Discrete Filter2/1 -> MATLAB Function/2(tau_g), WSE Inputs/2  "WE_t"
  PitComT/1 -> Discrete Filter/1
  Soft Start/1(out) -> Switch/1
  Switch/1 -> v_hat/1
  HorWindV/1 -> MATLAB Function/11(HorWind), Discrete Filter3/1
  Constant4/1 -> Switch/2
  MATLAB Function/5(Debug) -> Demux1/1
  Demux1/1 -> Terminator1/1  "WE_Cp"
  Demux1/2 -> Terminator2/1  "WE_D"
  Clock1/1 -> MATLAB Function/10(t)
  Discrete Filter3/1 -> Switch/3
  NaN break/1(y) -> Soft Start/5(actual)

== system ROSCO/BldPitch Controller/Integral ==
  SpeedErr : Inport
  Gain : Inport  Port=2
  Min Pitch : Inport  Port=3
  Gain1 : Gain  Gain=simu.dt
  Maximum Pitch : Constant  Value=R.PC_MaxPit
  Minimum Pitch : Constant  Value=R.PC_MinPit
  Multiply : Product
  Saturate Integral Term : simulink/Discontinuities/Saturation Dynamic  OutMin=[]  OutMax=[]  OutDataTypeStr=Inherit: Same as second input  OutDataType=fixdt(1, 16)  OutScaling=2^-10  RndMeth=Nearest  DoSatur=off
  Sum : Sum  Inputs=|++
  Unit Delay : UnitDelay  SampleTime=-1  HasFrameUpgradeWarning=on
  IntSpdErr : Outport  VectorParamsAs1DForOutWhenUnconnected=off
  wires:
  Maximum Pitch/1 -> Saturate Integral Term/1
  Unit Delay/1 -> Sum/2
  Sum/1 -> Saturate Integral Term/2
  SpeedErr/1 -> Gain1/1
  Gain/1 -> Multiply/2
  Saturate Integral Term/1 -> IntSpdErr/1, Unit Delay/1
  Gain1/1 -> Multiply/1
  Multiply/1 -> Sum/1
  Min Pitch/1 -> Saturate Integral Term/3

== system ROSCO/Fl_PD/Integral ==
  x : Inport
  Gain : Inport  Port=2
  Gain1 : Gain  Gain=simu.dt
  Maximum Pitch : Constant  Value=100
  Minimum Pitch : Constant  Value=-100
  Multiply : Product
  Saturate Integral Term : simulink/Discontinuities/Saturation Dynamic  OutMin=[]  OutMax=[]  OutDataTypeStr=Inherit: Same as second input  OutDataType=fixdt(1, 16)  OutScaling=2^-10  RndMeth=Nearest  DoSatur=off
  Scope : Scope  NumInputPorts=2
  Sum : Sum  Inputs=|++
  Unit Delay : UnitDelay  SampleTime=-1  HasFrameUpgradeWarning=on
  Int x : Outport  VectorParamsAs1DForOutWhenUnconnected=off
  wires:
  Maximum Pitch/1 -> Saturate Integral Term/1
  Unit Delay/1 -> Sum/2
  Minimum Pitch/1 -> Saturate Integral Term/3
  Sum/1 -> Saturate Integral Term/2
  x/1 -> Scope/1, Gain1/1
  Gain/1 -> Multiply/2
  Saturate Integral Term/1 -> Scope/2, Int x/1, Unit Delay/1
  Gain1/1 -> Multiply/1
  Multiply/1 -> Sum/1

== system ROSCO/LinearModel_Simulink/Extract Azimuth [deg] ==
  OutData : Inport
  Azimut : Scope  NumInputPorts=2
  Extract Azimuth : Fcn  Expr=u(strmatch('Azimuth',OutList))
  Extract RotSpeed : Fcn  Expr=u(strmatch('RotSpeed',OutList))
  Integrator : Integrator
  mod2pi : Fcn  Expr=rem(u, 2*pi)
  rad2deg : Gain  Gain=1/pi*180
  rpm2rad/s : Gain  Gain=pi/30
  Azimuth : Outport
  wires:
  OutData/1 -> Extract RotSpeed/1, Extract Azimuth/1
  rpm2rad/s/1 -> Integrator/1
  mod2pi/1 -> rad2deg/1
  Integrator/1 -> mod2pi/1
  rad2deg/1 -> Azimut/2, Azimuth/1
  Extract RotSpeed/1 -> rpm2rad/s/1
  Extract Azimuth/1 -> Azimut/1

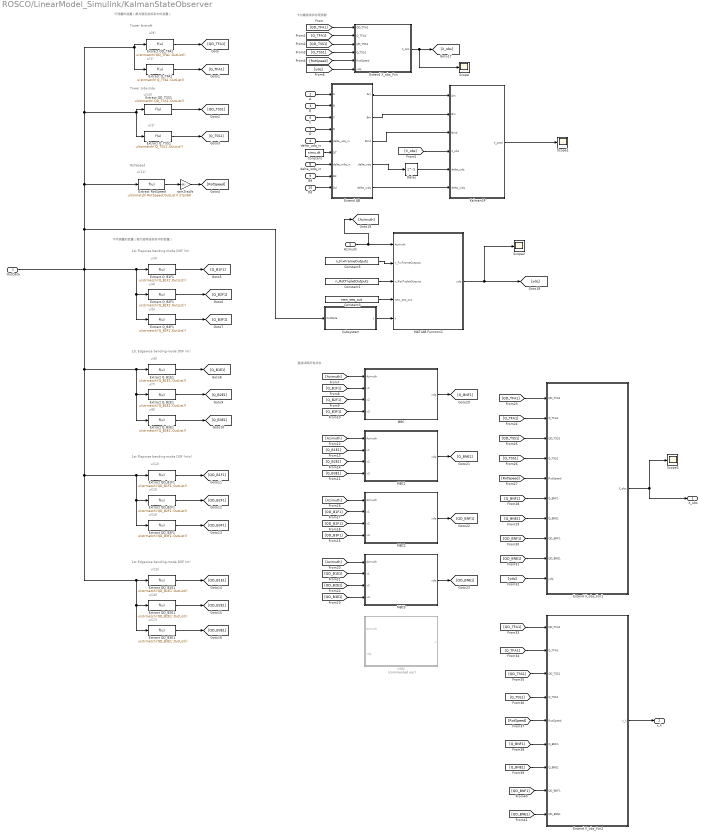
== system ROSCO/LinearModel_Simulink/KalmanStateObserver ==
  note: 直接读取所有状态
  note: u(11)
  note: u(2)
  note: u(10)
  note: u(1)
  note: u(9)
  note: 可测量的变量（都为固定坐标系中的变量）
  note: RotSpeed
  note: Tower fore-aft
  note: Tower side-side
  note: 卡尔曼滤波状态观测器
  note: 不可测量的变量（都为旋转坐标系中的变量）
  note: u(3)
  note: u(4)
  note: 1st Flapwise bending-mode DOF (m)
  note: u(5)
  note: u(6)
  note: u(7)
  note: 1st Edgewise bending-mode DOF (m)
  note: u(8)
  note: u(14)
  note: u(12)
  note: u(13)
  note: 1st Flapwise bending-mode DOF (m/s)
  note: 1st Edgewise bending-mode DOF (m)
  note: u(15)
  note: u(17)
  note: u(16)
  OutData : Inport
  A : Inport  Port=2
  B : Inport  Port=3
  delta_udq_in : Inport  Port=4
  Azimuth : Inport  Port=5
  C : Inport  Port=6
  D : Inport  Port=7
  delta_wdq_in : Inport  Port=8
  Bd : Inport  Port=9
  Dd : Inport  Port=10
  Constant : Constant  Value=simu.dt
  Constant1 : Constant  Value=n_RotTripletOutputs
  Constant3 : Constant  Value=new_seq_out
  Constant5 : Constant  Value=n_FixFrameOutputs
  Delay : Delay  DelayLength=1  InitialCondition=0
  Extend AB : MATLAB Function  TreatAsAtomicUnit=on
  Extend X_obs_Fcn : MATLAB Function  TreatAsAtomicUnit=on
  Extend X_obs_Fcn1 : MATLAB Function  TreatAsAtomicUnit=on
  Extend X_obs_Fcn2 : MATLAB Function  TreatAsAtomicUnit=on
  Extract QD_B1E1 : Fcn  Expr=u(strmatch('QD_B1E1',OutList))
  Extract QD_B1F1 : Fcn  Expr=u(strmatch('QD_B1F1',OutList))
  Extract QD_B2E1 : Fcn  Expr=u(strmatch('QD_B2E1',OutList))
  Extract QD_B2F1 : Fcn  Expr=u(strmatch('QD_B2F1',OutList))
  Extract QD_B3E1 : Fcn  Expr=u(strmatch('QD_B3E1',OutList))
  Extract QD_B3F1 : Fcn  Expr=u(strmatch('QD_B3F1',OutList))
  Extract QD_TFA1 : Fcn  Expr=u(strmatch('QD_TFA1',OutList))
  Extract QD_TSS1 : Fcn  Expr=u(strmatch('QD_TSS1',OutList))
  Extract Q_B1E1 : Fcn  Expr=u(strmatch('Q_B1E1',OutList))
  Extract Q_B1F1 : Fcn  Expr=u(strmatch('Q_B1F1',OutList))
  Extract Q_B2E1 : Fcn  Expr=u(strmatch('Q_B2E1',OutList))
  Extract Q_B2F1 : Fcn  Expr=u(strmatch('Q_B2F1',OutList))
  Extract Q_B3E1 : Fcn  Expr=u(strmatch('Q_B3E1',OutList))
  Extract Q_B3F1 : Fcn  Expr=u(strmatch('Q_B3F1',OutList))
  Extract Q_TFA1 : Fcn  Expr=u(strmatch('Q_TFA1',OutList))
  Extract Q_TSS1 : Fcn  Expr=u(strmatch('Q_TSS1',OutList))
  Extract RotSpeed : Fcn  Expr=u(strmatch('RotSpeed',OutList))
  KalmanSP : MATLAB Function  TreatAsAtomicUnit=on
  MATLAB Function1 : MATLAB Function  TreatAsAtomicUnit=on
  MBC : MATLAB Function  TreatAsAtomicUnit=on
  MBC1 : MATLAB Function  TreatAsAtomicUnit=on
  MBC2 : MATLAB Function  TreatAsAtomicUnit=on
  MBC3 : MATLAB Function  TreatAsAtomicUnit=on
  Scope{,1..3} (4 alike) : Scope
  Subsystem : Subsystem
  iMBC : MATLAB Function  Commented=on  TreatAsAtomicUnit=on
  rpm2rad/s : Gain  Gain=2*pi/60
  X_obs : Outport
  x_k : Outport  Port=2
  wires:
  Extract Q_TFA1/1 -> [Q_TFA1]
  Extract QD_TFA1/1 -> [QD_TFA1]
  Extract RotSpeed/1 -> rpm2rad/s/1
  rpm2rad/s/1 -> [RotSpeed]
  Extract QD_TSS1/1 -> [QD_TSS1]
  Extract Q_TSS1/1 -> [Q_TSS1]
  Extract Q_B1F1/1 -> [Q_B1F1]
  Extract Q_B2F1/1 -> [Q_B2F1]
  Extract Q_B3F1/1 -> [Q_B3F1]
  Extract Q_B3E1/1 -> [Q_B3E1]
  Extract Q_B2E1/1 -> [Q_B2E1]
  Extract Q_B1E1/1 -> [Q_B1E1]
  Extract QD_B3F1/1 -> [QD_B3F1]
  Extract QD_B1F1/1 -> [QD_B1F1]
  Extract QD_B2F1/1 -> [QD_B2F1]
  OutData/1 -> Extract QD_TFA1/1, Extract Q_TFA1/1, Extract QD_TSS1/1, Extract Q_TSS1/1, Extract RotSpeed/1, Subsystem/1(OutData), Extract QD_B1E1/1, Extract QD_B2E1/1, Extract QD_B3E1/1, Extract QD_B3F1/1, Extract QD_B2F1/1, Extract QD_B1F1/1, Extract Q_B1E1/1, Extract Q_B2E1/1, Extract Q_B3E1/1, Extract Q_B3F1/1, Extract Q_B2F1/1, Extract Q_B1F1/1
  Extract QD_B3E1/1 -> [QD_B3E1]
  Extract QD_B1E1/1 -> [QD_B1E1]
  Extract QD_B2E1/1 -> [QD_B2E1]
  [QD_TFA1] -> Extend X_obs_Fcn/1(QD_TFA1)
  [Q_TFA1] -> Extend X_obs_Fcn/2(Q_TFA1)
  [QD_TSS1] -> Extend X_obs_Fcn/3(QD_TSS1)
  [Q_TSS1] -> Extend X_obs_Fcn/4(Q_TSS1)
  [RotSpeed] -> Extend X_obs_Fcn/5(RotSpeed)
  Extend X_obs_Fcn/1(X_obs) -> Scope/1, [X_obs]
  [X_obs] -> KalmanSP/4(X_obs)
  Delay/1 -> KalmanSP/5(delta_udq)
  A/1 -> Extend AB/1(A)
  B/1 -> Extend AB/2(B)
  delta_udq_in/1 -> Extend AB/5(delta_udq_in)
  Extend AB/4(delta_udq) -> Delay/1
  Extend AB/2(Bm) -> KalmanSP/2(Bm)
  Extend AB/1(Am) -> KalmanSP/1(Am)
  C/1 -> Extend AB/3(C)
  D/1 -> Extend AB/4(D)
  KalmanSP/1(X_pred) -> Scope1/1
  Subsystem/1(y) -> MATLAB Function1/5(y)
  Constant5/1 -> MATLAB Function1/2(n_FixFrameOutputs)
  Constant1/1 -> MATLAB Function1/3(n_RotTripletOutputs)
  Constant3/1 -> MATLAB Function1/4(new_seq_out)
  Azimuth/1 -> [Azimuth], MATLAB Function1/1(Azimuth)
  MATLAB Function1/1(ydq) -> Scope2/1, [ydq]
  [ydq] -> Extend X_obs_Fcn/6(ydq)
  [Azimuth] -> MBC/1(Azimuth)
  [Q_B1F1] -> MBC/2(x1)
  [Q_B2F1] -> MBC/3(x2)
  [Q_B3F1] -> MBC/4(x3)
  [Q_B3E1] -> MBC1/4(x3)
  [Q_B2E1] -> MBC1/3(x2)
  [Q_B1E1] -> MBC1/2(x1)
  [Azimuth] -> MBC1/1(Azimuth)
  [Azimuth] -> MBC2/1(Azimuth)
  [QD_B1F1] -> MBC2/2(x1)
  [QD_B2F1] -> MBC2/3(x2)
  [QD_B3F1] -> MBC2/4(x3)
  [QD_B3E1] -> MBC3/4(x3)
  [QD_B2E1] -> MBC3/3(x2)
  [QD_B1E1] -> MBC3/2(x1)
  [Azimuth] -> MBC3/1(Azimuth)
  MBC/1(xdq) -> [Q_BNF1]
  MBC1/1(xdq) -> [Q_BNE1]
  MBC2/1(xdq) -> [QD_BNF1]
  MBC3/1(xdq) -> [QD_BNE1]
  [Q_TFA1] -> Extend X_obs_Fcn1/2(Q_TFA1)
  [QD_TSS1] -> Extend X_obs_Fcn1/3(QD_TSS1)
  [RotSpeed] -> Extend X_obs_Fcn1/5(RotSpeed)
  [QD_TFA1] -> Extend X_obs_Fcn1/1(QD_TFA1)
  [Q_TSS1] -> Extend X_obs_Fcn1/4(Q_TSS1)
  [Q_BNF1] -> Extend X_obs_Fcn1/6(Q_BNF1)
  [Q_BNE1] -> Extend X_obs_Fcn1/7(Q_BNE1)
  [QD_BNF1] -> Extend X_obs_Fcn1/8(QD_BNF1)
  [QD_BNE1] -> Extend X_obs_Fcn1/9(QD_BNE1)
  [ydq] -> Extend X_obs_Fcn1/10(ydq)
  Extend X_obs_Fcn1/1(X_obs) -> Scope3/1, X_obs/1
  [QD_TSS1] -> Extend X_obs_Fcn2/3(QD_TSS1)
  [QD_TFA1] -> Extend X_obs_Fcn2/1(QD_TFA1)
  [Q_TSS1] -> Extend X_obs_Fcn2/4(Q_TSS1)
  [QD_BNE1] -> Extend X_obs_Fcn2/9(QD_BNE1)
  [Q_TFA1] -> Extend X_obs_Fcn2/2(Q_TFA1)
  [RotSpeed] -> Extend X_obs_Fcn2/5(RotSpeed)
  [Q_BNF1] -> Extend X_obs_Fcn2/6(Q_BNF1)
  [QD_BNF1] -> Extend X_obs_Fcn2/8(QD_BNF1)
  [Q_BNE1] -> Extend X_obs_Fcn2/7(Q_BNE1)
  Extend X_obs_Fcn2/1(x_k) -> x_k/1
  Constant/1 -> Extend AB/6(DT)
  delta_wdq_in/1 -> Extend AB/7(delta_wdq_in)
  Bd/1 -> Extend AB/8(Bd)
  Dd/1 -> Extend AB/9(Dd)
  Extend AB/3(Bmd) -> KalmanSP/3(Bmd)
  Extend AB/5(delta_wdq) -> KalmanSP/6(delta_wdq)

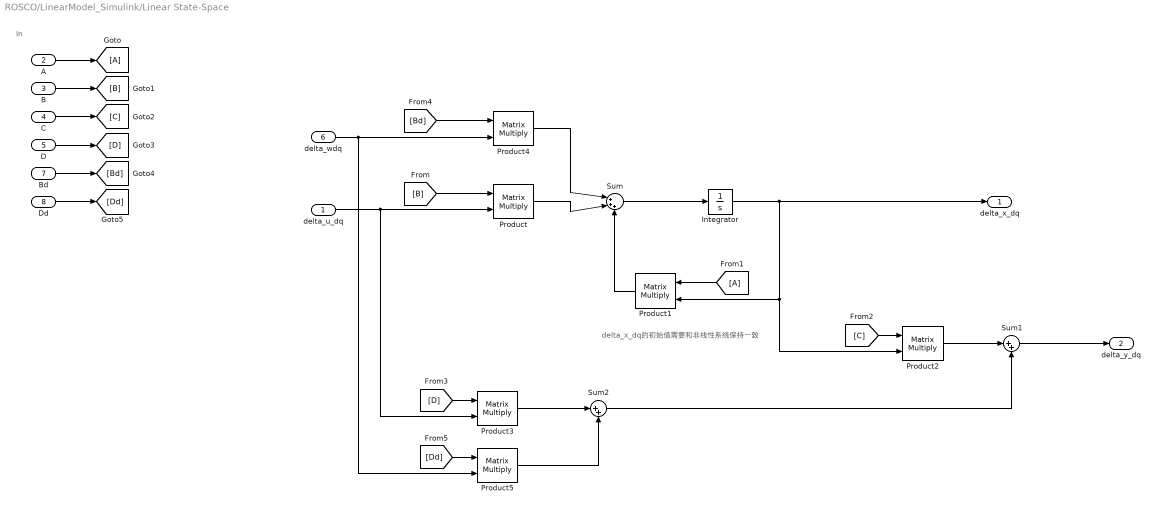
== system ROSCO/LinearModel_Simulink/Linear State-Space ==
  note: In
  note: delta_x_dq的初始值需要和非线性系统保持一致
  delta_u_dq : Inport
  A : Inport  Port=2
  B : Inport  Port=3
  C : Inport  Port=4
  D : Inport  Port=5
  delta_wdq : Inport  Port=6
  Bd : Inport  Port=7
  Dd : Inport  Port=8
  From1 : From
  Goto : Goto
  Integrator : Integrator
  Product{,1..5} (6 alike) : Product  Multiplication=Matrix(*)
  Sum : Sum  Inputs=|+++
  Sum1 : Sum  Inputs=|++
  Sum2 : Sum  Inputs=|++
  delta_x_dq : Outport
  delta_y_dq : Outport  Port=2
  wires:
  delta_u_dq/1 -> Product3/2, Product/2
  Sum/1 -> Integrator/1
  Integrator/1 -> Product2/2, Product1/2, delta_x_dq/1
  Product2/1 -> Sum1/1
  [B] -> Product/1
  From1/1 -> Product1/1
  [C] -> Product2/1
  [D] -> Product3/1
  A/1 -> Goto/1
  B/1 -> [B]
  C/1 -> [C]
  D/1 -> [D]
  Sum1/1 -> delta_y_dq/1
  Bd/1 -> [Bd]
  Dd/1 -> [Dd]
  Product1/1 -> Sum/3
  Product/1 -> Sum/2
  [Bd] -> Product4/1
  delta_wdq/1 -> Product5/2, Product4/2
  Product4/1 -> Sum/1
  Product3/1 -> Sum2/1
  Sum2/1 -> Sum1/2
  [Dd] -> Product5/1
  Product5/1 -> Sum2/2

== system ROSCO/LinearModel_Simulink/Subsystem ==
  Azimuth : Inport
  xop : Inport  Port=2
  Constant1 : Constant  Value=new_seq_states
  Constant7 : Constant  Value=n_FixFrameStates2
  Constant8 : Constant  Value=n_RotTripletStates2
  MATLAB Function1 : MATLAB Function  TreatAsAtomicUnit=on
  xop_dq : Outport
  wires:
  Constant1/1 -> MATLAB Function1/5(new_seq_inp)
  Constant7/1 -> MATLAB Function1/2(n_FixFrameInputs)
  xop/1 -> MATLAB Function1/4(xop)
  Azimuth/1 -> MATLAB Function1/1(Azimuth)
  MATLAB Function1/1(xop_dq) -> xop_dq/1
  Constant8/1 -> MATLAB Function1/3(n_RotTripletInputs)

== system ROSCO/LinearModel_Simulink/Subsystem1 ==
  Azimuth : Inport
  delta_y_dq : Inport  Port=2
  Constant5 : Constant  Value=n_RotTripletOutputs
  Constant6 : Constant  Value=new_seq_out
  Constant7 : Constant  Value=n_FixFrameOutputs
  MATLAB Function1 : MATLAB Function  TreatAsAtomicUnit=on
  delta_y : Outport
  wires:
  Constant6/1 -> MATLAB Function1/4(new_seq_out)
  Azimuth/1 -> MATLAB Function1/1(Azimuth)
  Constant5/1 -> MATLAB Function1/3(n_RotTripletOutputs)
  delta_y_dq/1 -> MATLAB Function1/5(y_dq)
  MATLAB Function1/1(y) -> delta_y/1
  Constant7/1 -> MATLAB Function1/2(n_FixFrameOutputs)

== system ROSCO/LinearModel_Simulink/Subsystem2 ==
  Azimuth : Inport
  y_dq : Inport  Port=2
  Constant5 : Constant  Value=n_RotTripletOutputs
  Constant6 : Constant  Value=new_seq_out
  Constant7 : Constant  Value=n_FixFrameOutputs
  MATLAB Function1 : MATLAB Function  TreatAsAtomicUnit=on
  y : Outport
  wires:
  Constant6/1 -> MATLAB Function1/4(new_seq_out)
  Azimuth/1 -> MATLAB Function1/1(Azimuth)
  Constant5/1 -> MATLAB Function1/3(n_RotTripletOutputs)
  y_dq/1 -> MATLAB Function1/5(y_dq)
  MATLAB Function1/1(y) -> y/1
  Constant7/1 -> MATLAB Function1/2(n_FixFrameOutputs)

== system ROSCO/LinearModel_Simulink/Switch op under Azimuth ==
  Azimuth : Inport
  delta_xdq : Inport  Port=2
  yop_list : Inport  Port=3
  xop : Inport  Port=4
  Integrator : Integrator
  Scope : Scope
  Select delta_wg : Fcn  Expr=u(11)
  Select wg : Fcn  Expr=u(11)
  Sum2 : Sum  Inputs=|++
  Switch op under Azimuth : MATLAB Function  TreatAsAtomicUnit=on
  "[deg]" : Constant  Value=Azimuth_list
  mod2pi : Fcn  Expr=rem(u, 2*pi)
  rad2deg : Gain  Gain=1/pi*180
  yop : Outport
  Azimuth_out : Outport  Port=2
  wires:
  "[deg]"/1 -> Switch op under Azimuth/2(Azimuth_list)
  Switch op under Azimuth/1(yop) -> yop/1
  Azimuth/1 -> Switch op under Azimuth/1(Azimuth)
  yop_list/1 -> Switch op under Azimuth/3(yop_36)
  rad2deg/1 -> Azimuth_out/1
  mod2pi/1 -> rad2deg/1
  Integrator/1 -> mod2pi/1
  Sum2/1 -> Integrator/1, Scope/1
  xop/1 -> Select wg/1
  delta_xdq/1 -> Select delta_wg/1
  Select delta_wg/1 -> Sum2/2
  Select wg/1 -> Sum2/1

== system ROSCO/LinearModel_Simulink/SwitchOP ==
  WindSpeed : Inport
  MATLAB Function : MATLAB Function  TreatAsAtomicUnit=on
  A : Outport
  B : Outport  Port=2
  C : Outport  Port=3
  D : Outport  Port=4
  yop_list : Outport  Port=5
  xop : Outport  Port=6
  uop : Outport  Port=7
  Bd : Outport  Port=8
  Dd : Outport  Port=9
  wop : Outport  Port=10
  wires:
  WindSpeed/1 -> MATLAB Function/1(windspeed)
  MATLAB Function/1(A) -> A/1
  MATLAB Function/2(B) -> B/1
  MATLAB Function/3(C) -> C/1
  MATLAB Function/4(D) -> D/1
  MATLAB Function/7(yop_list) -> yop_list/1
  MATLAB Function/8(xop) -> xop/1
  MATLAB Function/9(uop) -> uop/1
  MATLAB Function/5(Bd) -> Bd/1
  MATLAB Function/6(Dd) -> Dd/1
  MATLAB Function/10(wop) -> wop/1
